simulink model "DW_RTK_Simulink_Model"  (R2022b)
settings: Solver=VariableStepAuto  StartTime=0.0  StopTime=10.0  RelTol=1e-3
settings Model: Creator=HP  LastModifiedBy=HP

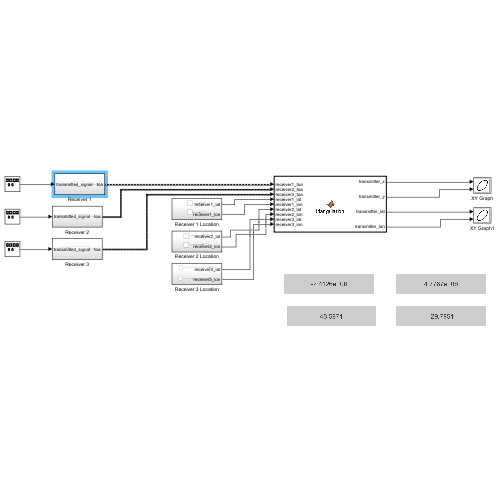
[thumbnail: Simulink's stored preview of the top-level diagram]
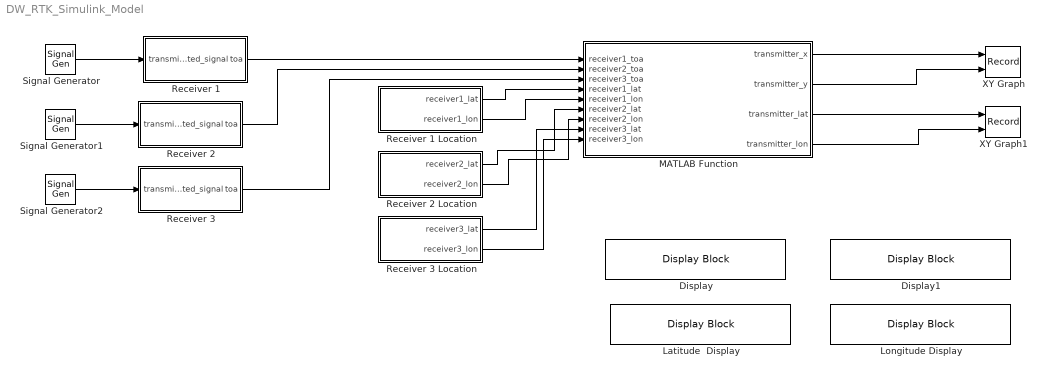
== system DW_RTK_Simulink_Model ==
  Display : DisplayBlock  LabelPosition=Hide  Transparency=1
  Display1 : DisplayBlock  LabelPosition=Hide  Transparency=1
  Latitude  Display : DisplayBlock  LabelPosition=Hide  Transparency=1
  Longitude Display : DisplayBlock  LabelPosition=Hide  Transparency=1
  MATLAB Function : MATLAB Function  TreatAsAtomicUnit=on
  Receiver 1 : Subsystem
  Receiver 1 Location : Subsystem
  Receiver 2 : Subsystem
  Receiver 2 Location : Subsystem
  Receiver 3 : Subsystem
  Receiver 3 Location : Subsystem
  Signal Generator : SignalGenerator  WaveForm=square  Amplitude=50  Frequency=50
  Signal Generator1 : SignalGenerator  WaveForm=square  Amplitude=50  Frequency=50
  Signal Generator2 : SignalGenerator  WaveForm=square  Amplitude=50  Frequency=50
  XY Graph : Record  FileSettingsInternal="{\"entries\":[{\"content\":{\"excelSettings\":{\"content\":{},\"type\":\"Streamout.ExcelSettings\"}},\"type\":\"Streamout.FileSettingStorage\",\"uuid\":\"78f437fe-cc33-4711-991f-d5d90419eef6\"}],\"packageUris\":[\"http://schema.mathworks.com/mf0/streamout_blocks/R2020a\"],\"version\":\"1.0\"}"  Layout=[1 1]  SignalsInternal="{\"entries\":[{\"content\":{\"signals\":[{\"content\":{\"blockPath\":[\"RADIO_TRIAN/XY Graph\"],\"channel\":[],\"dimensions\":[1],\"domain\":\"RADIO_TRIAN/XY Graph\",\"lineColor\":\"#a2142f\",\"plots\":[1],\"port\":1,\"sid\":[],\"signalID\":16,\"signalName\":\"MATLAB Function:1\"},\"type\":\"RecordBlkView.Signal\",\"uuid\":\"aec5dcd8-38c0-4d1e-bb55-593fe99361f8\"},{\"content\":{\"blockPath\":[\"RADIO_TRIAN/XY Graph\"],\"channel\":[],\"dimensions\":[1],\"domain\":\"RADIO_TRIAN/XY Graph\",\"lineColor\":\"#139fff\",\"plots\":[1],\"port\":2,\"sid\":[],\"signalID\":19,\"signalName\":\"MATLAB Function:2\"},\"type\":\"RecordBlkView.Signal\",\"uuid\":\"7964030e-2f3a-40d2-b0aa-92a7b022d92f\"}]},\"type\":\"RecordBlkView.InputSignals\",\"uuid\":\"53a57b4a-5bc8-472a-8458-a9e816b27812\"}],\"packageUris\":[\"http://schema.mathworks.com/mf0/streamout_blocks/R2020a\"],\"version\":\"1.0\"}"  VisualizationBindings="{\"xyplotplugin\":{\"info\":[{\"series\":[{\"bindingParametersList\":[{\"parameter\":\"X-Axis\",\"signalID\":16,\"signalName\":\"MATLAB Function:1\"},{\"parameter\":\"Y-Axis\",\"signalID\":19,\"signalName\":\"MATLAB Function:2\"}],\"seriesID\":56204}],\"subplotID\":1}]}}"  CompatibilityTag=XY
  XY Graph1 : Record  FileSettingsInternal="{\"entries\":[{\"content\":{\"excelSettings\":{\"content\":{},\"type\":\"Streamout.ExcelSettings\"}},\"type\":\"Streamout.FileSettingStorage\",\"uuid\":\"a9c0d6e3-eeaa-49d8-b273-48d49146e6df\"}],\"packageUris\":[\"http://schema.mathworks.com/mf0/streamout_blocks/R2020a\"],\"version\":\"1.0\"}"  Layout=[1 1]  SignalsInternal="{\"entries\":[{\"content\":{\"signals\":[{\"content\":{\"blockPath\":[\"RADIO_TRIAN/XY Graph1\"],\"channel\":[],\"dimensions\":[1],\"domain\":\"RADIO_TRIAN/XY Graph1\",\"lineColor\":\"#a2142f\",\"plots\":[1],\"port\":1,\"sid\":[],\"signalID\":8,\"signalName\":\"MATLAB Function:3\"},\"type\":\"RecordBlkView.Signal\",\"uuid\":\"d9f36468-47d4-4939-b37d-3467dd770d02\"},{\"content\":{\"blockPath\":[\"RADIO_TRIAN/XY Graph1\"],\"channel\":[],\"dimensions\":[1],\"domain\":\"RADIO_TRIAN/XY Graph1\",\"lineColor\":\"#139fff\",\"plots\":[1],\"port\":2,\"sid\":[],\"signalID\":11,\"signalName\":\"MATLAB Function:4\"},\"type\":\"RecordBlkView.Signal\",\"uuid\":\"259d8c55-5a7d-46d2-b28a-aa8d3790f783\"}]},\"type\":\"RecordBlkView.InputSignals\",\"uuid\":\"6c35f51f-bb8e-4a95-969a-4ccfb8ea9555\"}],\"packageUris\":[\"http://schema.mathworks.com/mf0/streamout_blocks/R2020a\"],\"version\":\"1.0\"}"  VisualizationBindings="{\"xyplotplugin\":{\"info\":[{\"series\":[{\"bindingParametersList\":[{\"parameter\":\"X-Axis\",\"signalID\":8,\"signalName\":\"MATLAB Function:3\"},{\"parameter\":\"Y-Axis\",\"signalID\":11,\"signalName\":\"MATLAB Function:4\"}],\"seriesID\":43683}],\"subplotID\":1}]}}"  CompatibilityTag=XY
  wires:
  Receiver 1/1(toa) -> MATLAB Function/1(receiver1_toa)
  Receiver 2/1(toa) -> MATLAB Function/2(receiver2_toa)
  Receiver 3/1(toa) -> MATLAB Function/3(receiver3_toa)
  Receiver 1 Location/1(receiver1_lat) -> MATLAB Function/4(receiver1_lat)
  Receiver 1 Location/2(receiver1_lon) -> MATLAB Function/5(receiver1_lon)
  Receiver 2 Location/1(receiver2_lat) -> MATLAB Function/6(receiver2_lat)
  Receiver 2 Location/2(receiver2_lon) -> MATLAB Function/7(receiver2_lon)
  Receiver 3 Location/1(receiver3_lat) -> MATLAB Function/8(receiver3_lat)
  Receiver 3 Location/2(receiver3_lon) -> MATLAB Function/9(receiver3_lon)
  Signal Generator/1 -> Receiver 1/1(transmitted_signal)
  Signal Generator1/1 -> Receiver 2/1(transmitted_signal)
  Signal Generator2/1 -> Receiver 3/1(transmitted_signal)
  MATLAB Function/1(transmitter_x) -> XY Graph/1
  MATLAB Function/2(transmitter_y) -> XY Graph/2
  MATLAB Function/3(transmitter_lat) -> XY Graph1/1
  MATLAB Function/4(transmitter_lon) -> XY Graph1/2

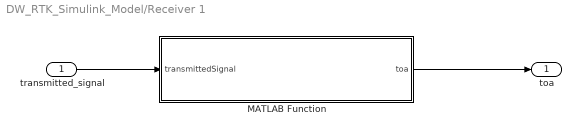
== system DW_RTK_Simulink_Model/Receiver 1 ==
  transmitted_signal : Inport
  MATLAB Function : MATLAB Function  TreatAsAtomicUnit=on  SystemSampleTime=10000
  toa : Outport
  wires:
  transmitted_signal/1 -> MATLAB Function/1(transmittedSignal)
  MATLAB Function/1(toa) -> toa/1

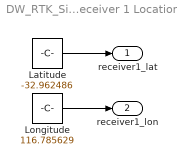
== system DW_RTK_Simulink_Model/Receiver 1 Location ==
  Latitude : Constant  Value=-32.962486
  Longitude : Constant  Value=116.785629
  receiver1_lat : Outport
  receiver1_lon : Outport  Port=2
  wires:
  Latitude/1 -> receiver1_lat/1
  Longitude/1 -> receiver1_lon/1

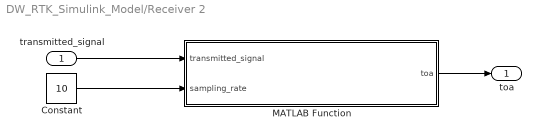
== system DW_RTK_Simulink_Model/Receiver 2 ==
  transmitted_signal : Inport
  Constant : Constant  Value=10
  MATLAB Function : MATLAB Function  TreatAsAtomicUnit=on  SystemSampleTime=10000
  toa : Outport
  wires:
  MATLAB Function/1(toa) -> toa/1
  transmitted_signal/1 -> MATLAB Function/1(transmitted_signal)
  Constant/1 -> MATLAB Function/2(sampling_rate)

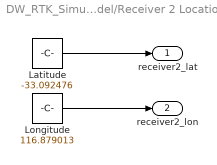
== system DW_RTK_Simulink_Model/Receiver 2 Location ==
  Latitude : Constant  Value=-33.092476
  Longitude : Constant  Value=116.879013
  receiver2_lat : Outport
  receiver2_lon : Outport  Port=2
  wires:
  Longitude/1 -> receiver2_lon/1
  Latitude/1 -> receiver2_lat/1

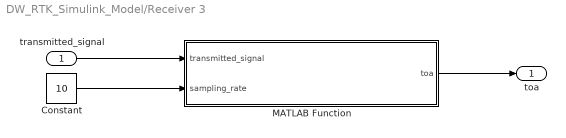
== system DW_RTK_Simulink_Model/Receiver 3 ==
  transmitted_signal : Inport
  Constant : Constant  Value=10
  MATLAB Function : MATLAB Function  TreatAsAtomicUnit=on  SystemSampleTime=10000
  toa : Outport
  wires:
  transmitted_signal/1 -> MATLAB Function/1(transmitted_signal)
  MATLAB Function/1(toa) -> toa/1
  Constant/1 -> MATLAB Function/2(sampling_rate)

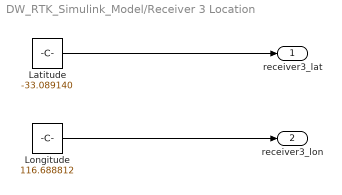
== system DW_RTK_Simulink_Model/Receiver 3 Location ==
  Latitude : Constant  Value=-33.089140
  Longitude : Constant  Value=116.688812
  receiver3_lat : Outport
  receiver3_lon : Outport  Port=2
  wires:
  Latitude/1 -> receiver3_lat/1
  Longitude/1 -> receiver3_lon/1

== matlab function DW_RTK_Simulink_Model/Receiver 2/MATLAB Function ==
  data: transmitted_signal input; toa output size=10000; sampling_rate input
function toa = calculateTOA_Receiver2(transmitted_signal, sampling_rate)
    % Generate random TOA values within a range (for demonstration purposes)
    % You can adjust the range and distribution based on your requirements
    min_toa = 0;  % Minimum TOA value
    max_toa = 10; % Maximum TOA value
    num_receivers = 3; % Number of receivers

    % Generate random TOA values for each receiver
    random_toa = (max_toa - min_toa) * rand(num_receivers, 1) + min_toa;
    
    % Select the TOA value for the current receiver
    toa = random_toa(1); % For Receiver 1
    
    % Ensure that TOA is fixed-size or specify upper bounds for variable-size
    toa = toa(1); % Select the first element to make it fixed-size
end

== matlab function DW_RTK_Simulink_Model/Receiver 1/MATLAB Function ==
  data toa settings: description=10000
  data: transmittedSignal input; toa output size=10000 [1..10000]
function toa = calculateTOA_Receiver1(transmittedSignal)
    % Generate random TOA values within a range (for demonstration purposes)
    % You can adjust the range and distribution based on your requirements
    min_toa = 0;  % Minimum TOA value
    max_toa = 10; % Maximum TOA value
    num_receivers = 3; % Number of receivers

    % Generate random TOA values for each receiver
    random_toa = (max_toa - min_toa) * rand(num_receivers, 1) + min_toa;
    
    % Select the TOA value for the current receiver
    toa = random_toa(1); % For Receiver 1
    
    % Ensure that TOA is fixed-size or specify upper bounds for variable-size
    toa = toa(1); % Select the first element to make it fixed-size
end

== matlab function DW_RTK_Simulink_Model/Receiver 3/MATLAB Function ==
  data: transmitted_signal input; toa output size=10000; sampling_rate input
function toa = calculateTOA_Receiver3(transmitted_signal, sampling_rate)
    % Generate random TOA values within a range (for demonstration purposes)
    % You can adjust the range and distribution based on your requirements
    min_toa = 0;  % Minimum TOA value
    max_toa = 10; % Maximum TOA value
    num_receivers = 3; % Number of receivers

    % Generate random TOA values for each receiver
    random_toa = (max_toa - min_toa) * rand(num_receivers, 1) + min_toa;
    
    % Select the TOA value for the current receiver
    toa = random_toa(1); % For Receiver 1
    
    % Ensure that TOA is fixed-size or specify upper bounds for variable-size
    toa = toa(1); % Select the first element to make it fixed-size
end

== matlab function DW_RTK_Simulink_Model/MATLAB Function ==
  data: receiver1_toa input; transmitter_x output; receiver2_toa input; receiver3_toa input; receiver1_lat input; receiver1_lon input; receiver2_lat input; receiver2_lon input; receiver3_lat input; receiver3_lon input; transmitter_y output; transmitter_lat output; transmitter_lon output
function [transmitter_x, transmitter_y, transmitter_lat, transmitter_lon] = triangulation(receiver1_toa, receiver2_toa, receiver3_toa, receiver1_lat, receiver1_lon, receiver2_lat, receiver2_lon, receiver3_lat, receiver3_lon)
    % Convert latitude and longitude coordinates to Cartesian coordinates (x, y)
    receiver1_location = latlon_to_cartesian(receiver1_lat, receiver1_lon);
    receiver2_location = latlon_to_cartesian(receiver2_lat, receiver2_lon);
    receiver3_location = latlon_to_cartesian(receiver3_lat, receiver3_lon);
    
    % Calculate distances between the transmitter and each receiver based on TOA
    % Assume speed of propagation (e.g., speed of light)
    speed_of_propagation = 299792458; % Speed of light in meters per second
    distance1 = receiver1_toa * speed_of_propagation;
    distance2 = receiver2_toa * speed_of_propagation;
    distance3 = receiver3_toa * speed_of_propagation;
    
    % Perform trilateration to estimate transmitter location
    transmitter_location = trilateration(receiver1_location, receiver2_location, receiver3_location, [distance1, distance2, distance3]);
   
    % Extract x and y coordinates
    transmitter_x = transmitter_location(1);
    transmitter_y = transmitter_location(2);
    
    % Convert Cartesian coordinates back to latitude and longitude
    [transmitter_lat, transmitter_lon] = cartesian_to_latlon(transmitter_x, transmitter_y);
end

function transmitter_location = trilateration(receiver1_location, receiver2_location, receiver3_location, distances)
    % Trilateration algorithm
    % Convert receiver locations to matrices
    P1 = receiver1_location(:)';
    P2 = receiver2_location(:)';
    P3 = receiver3_location(:)';
    
    % Calculate unit vectors from each receiver to the transmitter
    u1 = (P1 - P2) / norm(P1 - P2);
    u2 = (P1 - P3) / norm(P1 - P3);
    
    % Calculate transmitter location
    a = (distances(1)^2 - distances(2)^2 + norm(P2 - P1)^2) / (2 * norm(P2 - P1));
    b = (distances(1)^2 - distances(3)^2 + norm(P3 - P1)^2) / (2 * norm(P3 - P1));
    
    % Transmitter location in 2D (assuming z = 0)
    transmitter_location = P1 + a * u1 + b * u2;
end

function [latitude, longitude] = cartesian_to_latlon(x, y)
    % Convert Cartesian coordinates (x, y) to latitude and longitude
    % Assuming Earth is a perfect sphere for simplicity
    
    % Radius of the Earth (in meters)
    R = 6371000;
    
    % Calculate latitude and longitude
    lat_rad = asin(y / R);
    lon_rad = atan2(x, cos(lat_rad) * R);
    
    % Convert radians to degrees
    latitude = rad2deg(lat_rad);
    longitude = rad2deg(lon_rad);
end

function cartesian_location = latlon_to_cartesian(latitude, longitude)
    % Convert latitude and longitude coordinates to Cartesian coordinates (x, y)
    % Assuming Earth is a perfect sphere for simplicity
    
    % Radius of the Earth (in meters)
    R = 6371000;
    
    % Convert latitude and longitude to radians
    lat_rad = deg2rad(latitude);
    lon_rad = deg2rad(longitude);
    
    % Calculate Cartesian coordinates
    x = R * cos(lat_rad) * cos(lon_rad);
    y = R * cos(lat_rad) * sin(lon_rad);
    
    cartesian_location = [x, y];
end
